simulink model "LCC_pathprediction_2025b"  (R2025b)
settings: Solver=FixedStepDiscrete  StartTime=0.0  StopTime=700  FixedStep=.05  RelTol=1e-3
libraries: simulink x4, dspbuff3 x1
settings Model: Creator=scb548  LastModifiedBy=Sam Ball
settings OptimizationCC: ZeroExternalMemoryAtStartup=off  ZeroInternalMemoryAtStartup=off
settings RTWCC: SystemTargetFile=rtmaps.tlc  TemplateMakefile=rtmaps_default_tmf  PostCodeGenCommand=rtmaps_post_code_generation(buildInfo)  RetainRTWFile=on  TargetLang=C++  Description=Generate an RTMaps component embedding the model
settings STFCustomTargetCC: SystemTargetFile=rtmaps.tlc  TargetLangStandard=C++11 (ISO)  ModelReferenceCompliant=off  CombineOutputUpdateFcns=on  CodeInterfacePackaging=C++ class  SubcomponentCodeInterfacePackaging=C++ class  CPPClassGenCompliant=on  GRTInterface=off  RTMaps_MatFileLogging=0  RTMAPS_ARCH=x86_64  RTMaps_GenerateAllocFcn=0  RTMaps_IntegerCode=0  RTMaps_GRTInterface=0  RTMaps_CombineOutputUpdateFcns=1  RTMaps_MultiInstanceCode=1  DisplayOptimOptions=off  RTMAPS_OS=ubuntu2204  RTMaps_GenerateERTSFunction=0  RTMAPS_BOARD=ubuntu2204_x86_64  CustomFileTemplate=rtmaps_file_process.tlc  RTMAPS_SDKDIR=/opt/rtmaps
settings GRTTargetCC: TargetLangStandard=C++11 (ISO)  ModelReferenceCompliant=off  ParMdlRefBuildCompliant=off  CompOptLevelCompliant=off  MatFileLogging=off  CodeInterfacePackaging=C++ class  SubcomponentCodeInterfacePackaging=C++ class  UseToolchainInfoCompliant=off

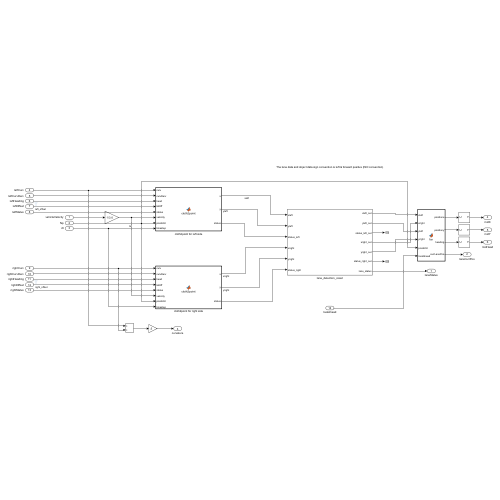
[thumbnail: Simulink's stored preview of the top-level diagram]
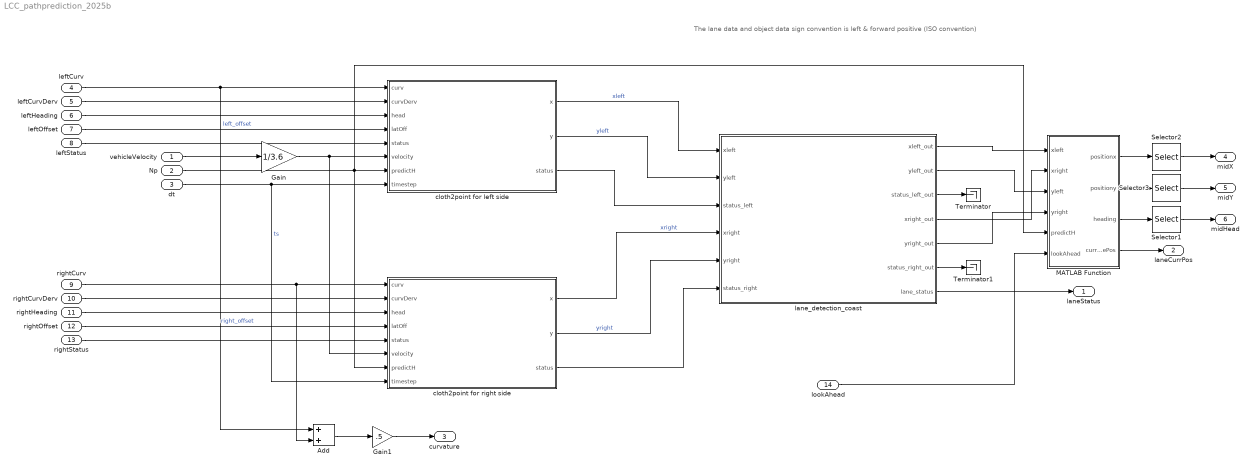
== system LCC_pathprediction_2025b ==
  note: The lane data and object data sign convention is left & forward positive (ISO convention)
  vehicleVelocity : Inport  OutDataTypeStr=double
  Np : Inport  Port=2
  dt : Inport  Port=3
  leftCurv : Inport  Port=4  OutDataTypeStr=double
  leftCurvDerv : Inport  Port=5  OutDataTypeStr=double
  leftHeading : Inport  Port=6  OutDataTypeStr=double
  leftOffset : Inport  Port=7
  leftStatus : Inport  Port=8  OutDataTypeStr=double
  rightCurv : Inport  Port=9  OutDataTypeStr=double
  rightCurvDerv : Inport  Port=10  OutDataTypeStr=double
  rightHeading : Inport  Port=11  OutDataTypeStr=double
  rightOffset : Inport  Port=12  OutDataTypeStr=double
  rightStatus : Inport  Port=13  OutDataTypeStr=double
  lookAhead : Inport  Port=14
  Add : Sum
  Gain : Gain  Gain=1/3.6
  Gain1 : Gain  Gain=.5
  MATLAB Function : MATLAB Function  TreatAsAtomicUnit=on
  Selector1 : Selector  InputPortWidth=30  IndexOptions=Index vector (dialog)  Indices=2  OutputSizes=1
  Selector2 : Selector  InputPortWidth=30  IndexOptions=Index vector (dialog)  Indices=2  OutputSizes=1
  Selector3 : Selector  InputPortWidth=30  IndexOptions=Index vector (dialog)  Indices=2  OutputSizes=1
  Terminator : Terminator
  Terminator1 : Terminator
  cloth2point for left side : MATLAB Function  TreatAsAtomicUnit=on
  cloth2point for right side : MATLAB Function  TreatAsAtomicUnit=on
  lane_detection_coast : Subsystem
  laneStatus : Outport
  laneCurrPos : Outport  Port=2
  curvature : Outport  Port=3
  midX : Outport  Port=4
  midY : Outport  Port=5
  midHead : Outport  Port=6
  wires:
  cloth2point for right side/2(y) -> lane_detection_coast/5(yright)  "yright"
  lane_detection_coast/6(status_right_out) -> Terminator1/1
  rightStatus/1 -> cloth2point for right side/5("status ")
  leftHeading/1 -> cloth2point for left side/3(head)
  Gain/1 -> cloth2point for left side/6(velocity), cloth2point for right side/6(velocity)
  MATLAB Function/3(heading) -> Selector1/1
  rightHeading/1 -> cloth2point for right side/3(head)
  Selector1/1 -> midHead/1
  MATLAB Function/1(positionx) -> Selector2/1
  lane_detection_coast/4(xright_out) -> MATLAB Function/2(xright)
  lane_detection_coast/1(xleft_out) -> MATLAB Function/1(xleft)
  leftCurvDerv/1 -> cloth2point for left side/2(curvDerv)
  MATLAB Function/4(currLanePos) -> laneCurrPos/1
  leftStatus/1 -> cloth2point for left side/5("status ")
  lane_detection_coast/3(status_left_out) -> Terminator/1
  vehicleVelocity/1 -> Gain/1
  Add/1 -> Gain1/1
  cloth2point for left side/1(x) -> lane_detection_coast/1(xleft)  "xleft"
  leftOffset/1 -> cloth2point for left side/4(latOff)  "left_offset"
  dt/1 -> cloth2point for left side/8(timestep), cloth2point for right side/8(timestep)  "ts"
  lane_detection_coast/5(yright_out) -> MATLAB Function/4(yright)
  Selector2/1 -> midX/1
  rightCurvDerv/1 -> cloth2point for right side/2(curvDerv)
  lane_detection_coast/2(yleft_out) -> MATLAB Function/3(yleft)
  MATLAB Function/2(positiony) -> Selector3/1
  Selector3/1 -> midY/1
  cloth2point for left side/2(y) -> lane_detection_coast/2(yleft)  "yleft"
  rightCurv/1 -> cloth2point for right side/1(curv), Add/2
  cloth2point for right side/3(status) -> lane_detection_coast/6(status_right)
  cloth2point for left side/3(status) -> lane_detection_coast/3(status_left)
  rightOffset/1 -> cloth2point for right side/4(latOff)  "right_offset"
  cloth2point for right side/1(x) -> lane_detection_coast/4(xright)  "xright"
  lane_detection_coast/7(lane_status) -> laneStatus/1
  Gain1/1 -> curvature/1
  Np/1 -> cloth2point for left side/7(predictH), cloth2point for right side/7(predictH), MATLAB Function/5(predictH)
  leftCurv/1 -> cloth2point for left side/1(curv), Add/1
  lookAhead/1 -> MATLAB Function/6(lookAhead)

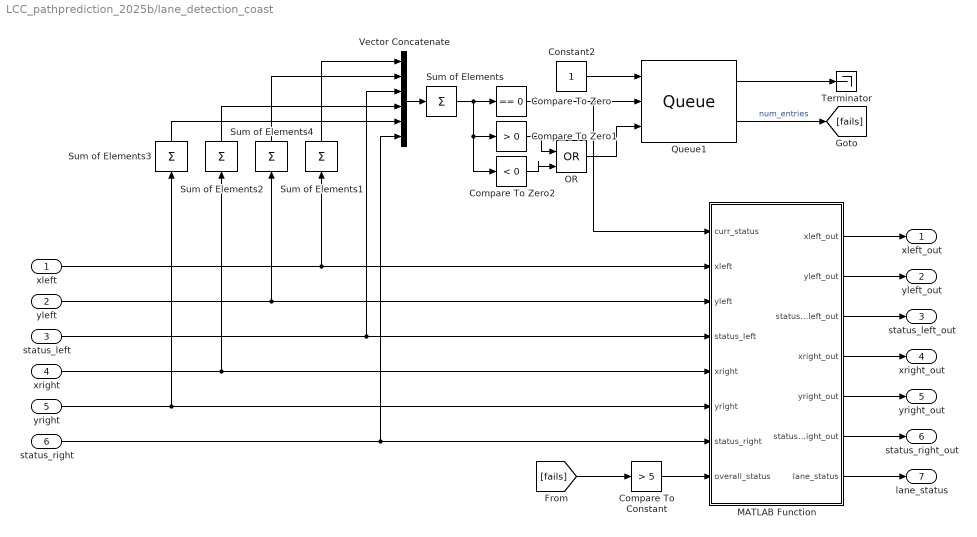
== system LCC_pathprediction_2025b/lane_detection_coast ==
  xleft : Inport  PortDimensions=[1 30]
  yleft : Inport  Port=2  PortDimensions=[1 30]
  status_left : Inport  Port=3  PortDimensions=1
  xright : Inport  Port=4  PortDimensions=[1 30]
  yright : Inport  Port=5  PortDimensions=[1 30]
  status_right : Inport  Port=6  PortDimensions=1
  Compare To Constant : simulink/Logic and Bit Operations/Compare To Constant  relop=>  const=5  OutDataTypeStr=boolean
  Compare To Zero : simulink/Logic and Bit Operations/Compare To Zero  relop===  OutDataTypeStr=boolean
  Compare To Zero1 : simulink/Logic and Bit Operations/Compare To Zero  relop=>  OutDataTypeStr=boolean
  Compare To Zero2 : simulink/Logic and Bit Operations/Compare To Zero  relop=<  OutDataTypeStr=boolean
  Constant2 : Constant  OutDataTypeStr=uint8
  MATLAB Function : MATLAB Function  TreatAsAtomicUnit=on
  OR : Logic  Operator=OR  IconShape=distinctive  AllPortsSameDT=off  OutDataTypeStr=boolean
  Queue1 : dspbuff3/Queue  depth=7  trigger=Non-zero sample  overflow=Ignore  pes=Ignore  eso=off  fso=off  nso=on  clr=off  clrOutport=off  adf=on
  Sum of Elements{,1..4} (5 alike) : Sum  Inputs=+
  Terminator : Terminator
  Vector Concatenate : Concatenate  NumInputs=6
  xleft_out : Outport  PortDimensions=[1 30]
  yleft_out : Outport  Port=2  PortDimensions=[1 30]
  status_left_out : Outport  Port=3  PortDimensions=1
  xright_out : Outport  Port=4  PortDimensions=[1 30]
  yright_out : Outport  Port=5  PortDimensions=[1 30]
  status_right_out : Outport  Port=6  PortDimensions=1
  lane_status : Outport  Port=7  PortDimensions=1
  wires:
  Queue1/1 -> Terminator/1
  Constant2/1 -> Queue1/1
  Queue1/2 -> [fails]  "num_entries"
  xleft/1 -> Sum of Elements1/1, MATLAB Function/2(xleft)
  yleft/1 -> Sum of Elements4/1, MATLAB Function/3(yleft)
  status_left/1 -> Vector Concatenate/3, MATLAB Function/4(status_left)
  xright/1 -> MATLAB Function/5(xright), Sum of Elements2/1
  yright/1 -> MATLAB Function/6(yright), Sum of Elements3/1
  status_right/1 -> Vector Concatenate/6, MATLAB Function/7(status_right)
  Vector Concatenate/1 -> Sum of Elements/1
  Sum of Elements/1 -> Compare To Zero2/1, Compare To Zero1/1, Compare To Zero/1
  Compare To Zero/1 -> Queue1/2, MATLAB Function/1(curr_status)
  Compare To Zero1/1 -> OR/1
  Compare To Zero2/1 -> OR/2
  OR/1 -> Queue1/3
  [fails] -> Compare To Constant/1
  MATLAB Function/1(xleft_out) -> xleft_out/1
  MATLAB Function/2(yleft_out) -> yleft_out/1
  MATLAB Function/3(status_left_out) -> status_left_out/1
  MATLAB Function/4(xright_out) -> xright_out/1
  MATLAB Function/5(yright_out) -> yright_out/1
  MATLAB Function/6(status_right_out) -> status_right_out/1
  MATLAB Function/7(lane_status) -> lane_status/1
  Sum of Elements1/1 -> Vector Concatenate/1
  Sum of Elements2/1 -> Vector Concatenate/4
  Sum of Elements3/1 -> Vector Concatenate/5
  Sum of Elements4/1 -> Vector Concatenate/2
  Compare To Constant/1 -> MATLAB Function/8(overall_status)

== matlab function LCC_pathprediction_2025b/lane_detection_coast/MATLAB Function ==
  data: curr_status input; xleft input size=[1 30]; xleft_out output size=[1 30]; yleft input size=[1 30]; status_left input; xright input size=[1 30]; yright input size=[1 30]; status_right input; yleft_out output size=[1 30]; status_left_out output; xright_out output size=[1 30]; yright_out output size=[1 30]; status_right_out output; overall_status input; lane_status output
function [xleft_out, yleft_out, status_left_out, xright_out, yright_out, status_right_out, lane_status] = ...
    fcn(curr_status, xleft, yleft, status_left, xright, yright, status_right, overall_status)

% Declare and set persistant variables
persistent xleft_prev yleft_prev status_left_prev xright_prev yright_prev status_right_prev

if isempty(xleft_prev)
    xleft_prev = xleft;
    yleft_prev = yleft;
    status_left_prev = status_left;

    xright_prev = xright;
    yright_prev = yright;
    status_right_prev = status_right;
end

xleft_out = zeros(size(xleft_prev));
yleft_out = zeros(size(yleft_prev));
status_left_out = 0;

xright_out = zeros(size(xright_prev));
yright_out = zeros(size(yright_prev));
status_right_out = 0;

% Current status of the lane detection
lane_status = 1;

% if the signal is unavaliable, set all outputs to zero
if overall_status

    lane_status = 0;

    return
end

% Use prev signals if it is unavalaible for the timestep
if curr_status && ~overall_status
    xleft_out = xleft_prev;
    yleft_out = yleft_prev;
    status_left_out = status_left_prev;

    xright_out = xright_prev;
    yright_out = yright_prev;
    status_right_out = status_right_prev;

    return
end

% Use signals as normal if no abnormalities
if ~curr_status && ~overall_status
    xleft_out = xleft;
    yleft_out = yleft;
    status_left_out = status_left;

    xright_out = xright;
    yright_out = yright;
    status_right_out = status_right;

    xleft_prev = xleft;
    yleft_prev = yleft;
    status_left_prev = status_left;

    xright_prev = xright;
    yright_prev = yright;
    status_right_prev = status_right;

    return
end

== matlab function LCC_pathprediction_2025b/MATLAB Function ==
  data: xleft input double size=[1, 30]; positionx output double size=[1, 30]; positiony output double size=[1, 30]; xright input double size=[1, 30]; yleft input double size=[1, 30]; yright input double size=[1, 30]; heading output double size=[1, 30]; currLanePos output; predictH input; lookAhead input
function [positionx, positiony, heading, currLanePos] = fcn(xleft, xright, yleft, yright, predictH, lookAhead)

%% Matrix Declarations
heading = zeros(1, predictH+5);
middle = [(xleft + xright)./2; ((yleft + yright)./2)];

%% Heading Calculation
for i = 1:predictH+4
    heading(i+1) = atan2(middle(2,i+1)-middle(2,i), middle(1,i+1)-middle(1,i));
end


%% Outputs
positionx = middle(1,:);
positiony = middle(2,:);
currLanePos = double([heading(lookAhead), positiony(lookAhead)]);

== matlab function LCC_pathprediction_2025b/cloth2point for left side ==
  data: x output double size=[1, 30]; curv input; curvDerv input; head input; latOff input; status input; y output double size=[1, 30]; velocity input double; status output; predictH input; timestep input
function [x, y, status] = cloth2point(curv, curvDerv, head, latOff, status, velocity, predictH, timestep)

%% Martix Declaration
l = zeros(1, predictH+5);

%% Calculate longitudinal distance

% Only calulate if there is a read lane
if status
    for i = 1:predictH+5
        l(i) = ((velocity*timestep)) * (i-1);
    end
end

%% Outputs
x = l;
y = (1/6)*curv.*(l.^3) + (1/2)*curvDerv.*(l.^2) + head.*l + latOff;

% https://ieeexplore.ieee.org/document/6641084

== matlab function LCC_pathprediction_2025b/cloth2point for right side ==
  data: x output double size=[1, 30]; curv input; curvDerv input; head input; latOff input; status input; y output double size=[1, 30]; velocity input double; status output; predictH input; timestep input
function [x, y, status] = cloth2point(curv, curvDerv, head, latOff, status, velocity, predictH, timestep)

%% Martix Declaration
l = zeros(1, predictH+5);

%% Calculate longitudinal distance

% Only calulate if there is a read lane
if status
    for i = 1:predictH+5
        l(i) = ((velocity*timestep)) * (i-1);
    end
end

%% Outputs
x = l;
y = (1/6)*curv.*(l.^3) + (1/2)*curvDerv.*(l.^2) + head.*l + latOff;

% https://ieeexplore.ieee.org/document/6641084
